simulink model "torqueWalkingR2012b"  (Simulink 8.0)
settings: Solver=FixedStepDiscrete  StartTime=0.0  StopTime=Config.t_end  FixedStep=Config.t_step  RelTol=1e-3
InitFcn:
  | cd(fileparts(which(bdroot)));
  | initTorqueWalking;
StopFcn:
  | disp_early_termination
undefined symbols (not defined in the file or in its folder): biasVectorConstraint_feet, Config, ConstraintMatrix_feet, DiscIntNeverNeededParam, Gains, ROBOT_DOF, Sat
libraries: WBToolboxLibrary x114, simulink x2
(part 1 of 4)
settings Model: Creator=gnava  LastModifiedBy=mcharbonneau
settings DataIOCC: LimitDataPoints=off  SaveFormat=StructureWithTime
settings OptimizationCC: ExpressionDepthLimit=128
settings DebuggingCC: UnderspecifiedInitializationDetection=Simplified  MergeDetectMultiDrivingBlocksExec=error  SolverPrmCheckMsg=none  InheritedTsInSrcMsg=none  UnconnectedLineMsg=none  FrameProcessingCompatibilityMsg=error  StateNameClashWarn=none  SFUnexpectedBacktrackingDiag=error  SFNoUnconditionalDefaultTransitionDiag=error
settings HardwareCC: ProdBitPerPointer=64  ProdLargestAtomicFloat=Float  ProdIntDivRoundTo=Zero  ProdEndianess=LittleEndian  ProdHWDeviceType=Specified
settings ModelReferenceCC: PropagateSignalLabelsOutOfModel=on
settings CodeAppCC: CustomSymbolStrType=$N$R$M_T
settings GRTTargetCC: CodeReplacementLibrary=C99 (ISO)  GeneratePreprocessorConditionals=Use local settings

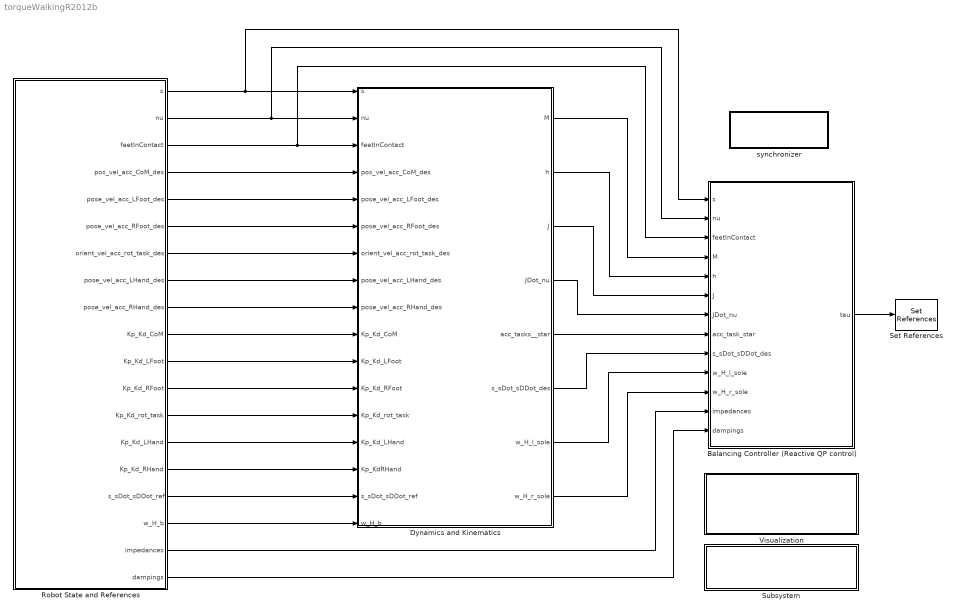
== system torqueWalkingR2012b ==
  Balancing Controller (Reactive QP control) : Subsystem
  Dynamics and Kinematics : Subsystem
  Robot State and References : Subsystem
  Set References : WBToolboxLibrary/wholeBodyActuators/Set References  controlType=Torque  fullOrSubControl=Full  controlledJoints=''  robotName=WBT_robotName  localName=WBT_modelName  wbiFile=WBT_wbiFilename  wbiList=WBT_wbiList
  Subsystem : Subsystem
      mask Display: disp('DATA FOR LEARNOPTIM_WBC')
  Visualization : Subsystem
      mask Display: disp('VISUALIZE AND DUMP DATA \n EARLY TERMINATION')
  synchronizer : Subsystem
      mask Display: disp('SYNCHRONIZER')
  wires:
  Robot State and References/2(nu) -> Dynamics and Kinematics/2(nu), Balancing Controller (Reactive QP control)/2(nu)
  Robot State and References/3(feetInContact) -> Dynamics and Kinematics/3(feetInContact), Balancing Controller (Reactive QP control)/3(feetInContact)
  Robot State and References/4(pos_vel_acc_CoM_des) -> Dynamics and Kinematics/4(pos_vel_acc_CoM_des)
  Robot State and References/5(pose_vel_acc_LFoot_des) -> Dynamics and Kinematics/5(pose_vel_acc_LFoot_des)
  Robot State and References/6(pose_vel_acc_RFoot_des) -> Dynamics and Kinematics/6(pose_vel_acc_RFoot_des)
  Robot State and References/11(Kp_Kd_LFoot) -> Dynamics and Kinematics/11(Kp_Kd_LFoot)
  Robot State and References/12(Kp_Kd_RFoot) -> Dynamics and Kinematics/12(Kp_Kd_RFoot)
  Robot State and References/13(Kp_Kd_rot_task) -> Dynamics and Kinematics/13(Kp_Kd_rot_task)
  Robot State and References/16(s_sDot_sDDot_ref) -> Dynamics and Kinematics/16(s_sDot_sDDot_ref)
  Robot State and References/17(w_H_b) -> Dynamics and Kinematics/17(w_H_b)
  Dynamics and Kinematics/4(JDot_nu) -> Balancing Controller (Reactive QP control)/7(JDot_nu)
  Robot State and References/1(s) -> Dynamics and Kinematics/1(s), Balancing Controller (Reactive QP control)/1(s)
  Dynamics and Kinematics/1(M) -> Balancing Controller (Reactive QP control)/4(M)
  Dynamics and Kinematics/2(h) -> Balancing Controller (Reactive QP control)/5(h)
  Dynamics and Kinematics/3(J) -> Balancing Controller (Reactive QP control)/6(J)
  Balancing Controller (Reactive QP control)/1(tau) -> Set References/1
  Dynamics and Kinematics/5(acc_tasks__star) -> Balancing Controller (Reactive QP control)/8(acc_task_star)
  Dynamics and Kinematics/6(s_sDot_sDDot_des) -> Balancing Controller (Reactive QP control)/9(s_sDot_sDDot_des)
  Dynamics and Kinematics/7(w_H_l_sole) -> Balancing Controller (Reactive QP control)/10(w_H_l_sole)
  Dynamics and Kinematics/8(w_H_r_sole) -> Balancing Controller (Reactive QP control)/11(w_H_r_sole)
  Robot State and References/18(impedances) -> Balancing Controller (Reactive QP control)/12(impedances)
  Robot State and References/19(dampings) -> Balancing Controller (Reactive QP control)/13(dampings)
  Robot State and References/15(Kp_Kd_RHand) -> Dynamics and Kinematics/15(Kp_KdRHand)
  Robot State and References/14(Kp_Kd_LHand) -> Dynamics and Kinematics/14(Kp_Kd_LHand)
  Robot State and References/8(pose_vel_acc_LHand_des) -> Dynamics and Kinematics/8(pose_vel_acc_LHand_des)
  Robot State and References/7(orient_vel_acc_rot_task_des) -> Dynamics and Kinematics/7(orient_vel_acc_rot_task_des)
  Robot State and References/9(pose_vel_acc_RHand_des) -> Dynamics and Kinematics/9(pose_vel_acc_RHand_des)
  Robot State and References/10(Kp_Kd_CoM) -> Dynamics and Kinematics/10(Kp_Kd_CoM)

== system torqueWalkingR2012b/Balancing Controller (Reactive QP control) ==
  s : Inport
  nu : Inport  Port=2
  feetInContact : Inport  Port=3
  M : Inport  Port=4
  h : Inport  Port=5
  J : Inport  Port=6
  JDot_nu : Inport  Port=7
  acc_task_star : Inport  Port=8
  s_sDot_sDDot_des : Inport  Port=9
  w_H_l_sole : Inport  Port=10
  w_H_r_sole : Inport  Port=11
  impedances : Inport  Port=12
  dampings : Inport  Port=13
  "   " : Constant  Value=ConstraintMatrix_feet
  "      " : Constant  Value=biasVectorConstraint_feet
  "             " : Selector  InputPortWidth=ROBOT_DOF+6  IndexOptions=Index vector (dialog)  Indices=[7:ROBOT_DOF+6]  OutputSizes=1
  Balancing Controller Function : MATLAB Function  TreatAsAtomicUnit=on
      settings: PermitHierarchicalResolution=ParametersOnly
  Compute joint torques (motor reflected inertia) : Subsystem
  Get Estimate : WBToolboxLibrary/wholeBodyStates/Get Estimate  estimateType=Joints Torque  robotName=WBT_robotName  localName=WBT_modelName  wbiFile=WBT_wbiFilename  wbiList=WBT_wbiList
  QPSolver (Reactive QP control) : Subsystem
  Saturation : Saturate  UpperLimit=Sat.tau_max  LowerLimit=-Sat.tau_max
  "holder " : WBToolboxLibrary/Utilities/holder 
  tau : Outport
  tag scope: exitFlagQP=global, f_LFoot=global, f_RFoot=global, tau=global, tau_des=global
  wires:
  QPSolver (Reactive QP control)/1(tau) -> Compute joint torques (motor reflected inertia)/1(invGamma*tau_motors)
  "holder "/1 -> QPSolver (Reactive QP control)/1(tau_0)
  Balancing Controller Function/3(ConstraintMatrix_equality) -> QPSolver (Reactive QP control)/5(ConstraintMatrix_equality)
  Balancing Controller Function/6(biasVectorConstraint_inequality) -> QPSolver (Reactive QP control)/8(biasVectorConstraint_inequality)
  Balancing Controller Function/2(gradient) -> QPSolver (Reactive QP control)/4(gradient)
  Balancing Controller Function/4(biasVectorConstraint_equality) -> QPSolver (Reactive QP control)/6(biasVectorConstraint_equality)
  Balancing Controller Function/5(ConstraintMatrix_inequality) -> QPSolver (Reactive QP control)/7(ConstraintMatrix_inequality)
  w_H_r_sole/1 -> Balancing Controller Function/15(w_H_r_sole)
  w_H_l_sole/1 -> Balancing Controller Function/14(w_H_l_sole)
  "      "/1 -> Balancing Controller Function/13(biasVectorConstraint_feet)
  "   "/1 -> Balancing Controller Function/12(ConstraintsMatrix_feet)
  s_sDot_sDDot_des/1 -> Balancing Controller Function/9(s_sDot_sDDot_des)
  nu/1 -> "             "/1
  s/1 -> Balancing Controller Function/7(s)
  dampings/1 -> Balancing Controller Function/6(dampings)
  impedances/1 -> Balancing Controller Function/5(impedances)
  h/1 -> Balancing Controller Function/3(h)
  M/1 -> Balancing Controller Function/2(M)
  Get Estimate/1 -> [tau], "holder "/1
  "             "/1 -> Balancing Controller Function/8(sDot)
  Saturation/1 -> tau/1, [tau_des]
  Balancing Controller Function/1(Hessian) -> QPSolver (Reactive QP control)/3(Hessian)
  feetInContact/1 -> QPSolver (Reactive QP control)/2(feetInContact), Balancing Controller Function/1(feetInContact)
  QPSolver (Reactive QP control)/2(f_LFoot) -> [f_LFoot]
  QPSolver (Reactive QP control)/3(f_RFoot) -> [f_RFoot]
  QPSolver (Reactive QP control)/4(exitFlagQP) -> [exitFlagQP]
  Compute joint torques (motor reflected inertia)/1(tau_joints) -> Saturation/1
  acc_task_star/1 -> Balancing Controller Function/10(acc_task_star)
  J/1 -> Balancing Controller Function/4(J)
  JDot_nu/1 -> Balancing Controller Function/11(JDot_nu)

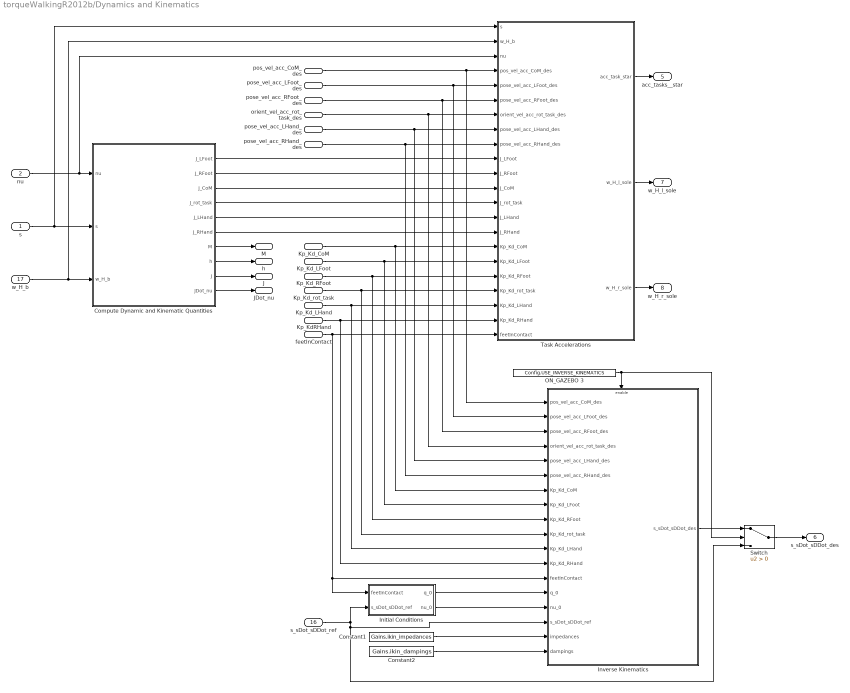
== system torqueWalkingR2012b/Dynamics and Kinematics ==
  s : Inport
  nu : Inport  Port=2
  feetInContact : Inport  Port=3
  pos_vel_acc_CoM_des : Inport  Port=4
  pose_vel_acc_LFoot_des : Inport  Port=5
  pose_vel_acc_RFoot_des : Inport  Port=6
  orient_vel_acc_rot_task_des : Inport  Port=7
  pose_vel_acc_LHand_des : Inport  Port=8
  pose_vel_acc_RHand_des : Inport  Port=9
  Kp_Kd_CoM : Inport  Port=10
  Kp_Kd_LFoot : Inport  Port=11
  Kp_Kd_RFoot : Inport  Port=12
  Kp_Kd_rot_task : Inport  Port=13
  Kp_Kd_LHand : Inport  Port=14
  Kp_KdRHand : Inport  Port=15
  s_sDot_sDDot_ref : Inport  Port=16
  w_H_b : Inport  Port=17
  Compute Dynamic and Kinematic Quantities : Subsystem
  Constant1 : Constant  Value=Gains.ikin_impedances
  Constant2 : Constant  Value=Gains.ikin_dampings
  Initial Conditions : Subsystem
  Inverse Kinematics : Subsystem
  ON_GAZEBO 3 : Constant  Value=Config.USE_INVERSE_KINEMATICS
  Switch : Switch  Criteria=u2 > Threshold
  Task Accelerations : Subsystem
  M : Outport
  h : Outport  Port=2
  J : Outport  Port=3
  JDot_nu : Outport  Port=4
  acc_tasks__star : Outport  Port=5
  s_sDot_sDDot_des : Outport  Port=6
  w_H_l_sole : Outport  Port=7
  w_H_r_sole : Outport  Port=8
  wires:
  pos_vel_acc_CoM_des/1 -> Inverse Kinematics/1(pos_vel_acc_CoM_des), Task Accelerations/4(pos_vel_acc_CoM_des)
  pose_vel_acc_LFoot_des/1 -> Inverse Kinematics/2(pose_vel_acc_LFoot_des), Task Accelerations/5(pose_vel_acc_LFoot_des)
  pose_vel_acc_RFoot_des/1 -> Inverse Kinematics/3(pose_vel_acc_RFoot_des), Task Accelerations/6(pose_vel_acc_RFoot_des)
  orient_vel_acc_rot_task_des/1 -> Inverse Kinematics/4(orient_vel_acc_rot_task_des), Task Accelerations/7(orient_vel_acc_rot_task_des)
  Kp_Kd_CoM/1 -> Inverse Kinematics/7(Kp_Kd_CoM), Task Accelerations/16(Kp_Kd_CoM)
  Kp_Kd_LFoot/1 -> Inverse Kinematics/8(Kp_Kd_LFoot), Task Accelerations/17(Kp_Kd_LFoot)
  Kp_Kd_RFoot/1 -> Inverse Kinematics/9(Kp_Kd_RFoot), Task Accelerations/18(Kp_Kd_RFoot)
  Kp_Kd_rot_task/1 -> Inverse Kinematics/10(Kp_Kd_rot_task), Task Accelerations/19(Kp_Kd_rot_task)
  Task Accelerations/1(acc_task_star) -> acc_tasks__star/1
  ON_GAZEBO 3/1 -> Switch/2, Inverse Kinematics/Enable
  Inverse Kinematics/1(s_sDot_sDDot_des) -> Switch/1
  nu/1 -> Task Accelerations/3(nu), Compute Dynamic and Kinematic Quantities/1(nu)
  s/1 -> Task Accelerations/1(s), Compute Dynamic and Kinematic Quantities/2(s)
  w_H_b/1 -> Task Accelerations/2(w_H_b), Compute Dynamic and Kinematic Quantities/3(w_H_b)
  Compute Dynamic and Kinematic Quantities/8(h) -> h/1
  Compute Dynamic and Kinematic Quantities/1(J_LFoot) -> Task Accelerations/10(J_LFoot)
  Compute Dynamic and Kinematic Quantities/2(J_RFoot) -> Task Accelerations/11(J_RFoot)
  Compute Dynamic and Kinematic Quantities/3(J_CoM) -> Task Accelerations/12(J_CoM)
  Compute Dynamic and Kinematic Quantities/7(M) -> M/1
  Compute Dynamic and Kinematic Quantities/4(J_rot_task) -> Task Accelerations/13(J_rot_task)
  Compute Dynamic and Kinematic Quantities/9(J) -> J/1
  Compute Dynamic and Kinematic Quantities/10(JDot_nu) -> JDot_nu/1
  s_sDot_sDDot_ref/1 -> Inverse Kinematics/16(s_sDot_sDDot_ref), Switch/3, Initial Conditions/2(s_sDot_sDDot_ref)
  Initial Conditions/1(q_0) -> Inverse Kinematics/14(q_0)
  Initial Conditions/2(nu_0) -> Inverse Kinematics/15(nu_0)
  Constant1/1 -> Inverse Kinematics/17(impedances)
  Constant2/1 -> Inverse Kinematics/18(dampings)
  Switch/1 -> s_sDot_sDDot_des/1
  feetInContact/1 -> Task Accelerations/22(feetInContact), Inverse Kinematics/13(feetInContact), Initial Conditions/1(feetInContact)
  Task Accelerations/2(w_H_l_sole) -> w_H_l_sole/1
  Task Accelerations/3(w_H_r_sole) -> w_H_r_sole/1
  Compute Dynamic and Kinematic Quantities/5(J_LHand) -> Task Accelerations/14(J_LHand)
  Compute Dynamic and Kinematic Quantities/6(J_RHand) -> Task Accelerations/15(J_RHand)
  pose_vel_acc_RHand_des/1 -> Inverse Kinematics/6(pose_vel_acc_RHand_des), Task Accelerations/9(pose_vel_acc_RHand_des)
  pose_vel_acc_LHand_des/1 -> Inverse Kinematics/5(pose_vel_acc_LHand_des), Task Accelerations/8(pose_vel_acc_LHand_des)
  Kp_Kd_LHand/1 -> Inverse Kinematics/11(Kp_Kd_LHand), Task Accelerations/20(Kp_Kd_LHand)
  Kp_KdRHand/1 -> Inverse Kinematics/12(Kp_Kd_RHand), Task Accelerations/21(Kp_Kd_RHand)

== system torqueWalkingR2012b/Robot State and References ==
  Gain Scheduling : Subsystem
  "Smooth References " : Subsystem
  State Machines : Subsystem
  s : Outport
  nu : Outport  Port=2
  feetInContact : Outport  Port=3
  pos_vel_acc_CoM_des : Outport  Port=4
  pose_vel_acc_LFoot_des : Outport  Port=5
  pose_vel_acc_RFoot_des : Outport  Port=6
  orient_vel_acc_rot_task_des : Outport  Port=7
  pose_vel_acc_LHand_des : Outport  Port=8
  pose_vel_acc_RHand_des : Outport  Port=9
  Kp_Kd_CoM : Outport  Port=10
  Kp_Kd_LFoot : Outport  Port=11
  Kp_Kd_RFoot : Outport  Port=12
  Kp_Kd_rot_task : Outport  Port=13
  Kp_Kd_LHand : Outport  Port=14
  Kp_Kd_RHand : Outport  Port=15
  s_sDot_sDDot_ref : Outport  Port=16
  w_H_b : Outport  Port=17
  impedances : Outport  Port=18
  dampings : Outport  Port=19
  wires:
  Gain Scheduling/1(Kp_Kd_CoM) -> Kp_Kd_CoM/1
  Gain Scheduling/2(Kp_Kd_LFoot) -> Kp_Kd_LFoot/1
  Gain Scheduling/3(Kp_Kd_RFoot) -> Kp_Kd_RFoot/1
  Gain Scheduling/4(Kp_Kd_rot_task) -> Kp_Kd_rot_task/1
  Gain Scheduling/7(impedances) -> impedances/1
  Gain Scheduling/8(dampings) -> dampings/1
  State Machines/5(state) -> Gain Scheduling/1(state), "Smooth References "/1(state)
  State Machines/4(feetInContact) -> feetInContact/1
  State Machines/3(nu) -> nu/1
  State Machines/2(w_H_b) -> w_H_b/1
  State Machines/8(references_CoM) -> "Smooth References "/4(references_CoM)
  State Machines/6(references_LFoot) -> "Smooth References "/2(references_LFoot)
  State Machines/7(references_RFoot) -> "Smooth References "/3(references_RFoot)
  State Machines/9(references_rot_task) -> "Smooth References "/5(references_rot_task)
  State Machines/12(references_s) -> "Smooth References "/8(references_s)
  "Smooth References "/1(pos_vel_acc_CoM_des) -> pos_vel_acc_CoM_des/1
  "Smooth References "/2(pose_vel_acc_LFoot_des) -> pose_vel_acc_LFoot_des/1
  "Smooth References "/3(pose_vel_acc_RFoot_des) -> pose_vel_acc_RFoot_des/1
  "Smooth References "/4(orient_vel_acc_rot_task_des) -> orient_vel_acc_rot_task_des/1
  "Smooth References "/7(s_sDot_sDDot_ref) -> s_sDot_sDDot_ref/1
  State Machines/1(s) -> s/1
  State Machines/10(references_LHand) -> "Smooth References "/6(references_LHand)
  State Machines/11(references_RHand) -> "Smooth References "/7(references_RHand)
  "Smooth References "/5(pose_vel_acc_LHand_des) -> pose_vel_acc_LHand_des/1
  "Smooth References "/6(pose_vel_acc_RHand_des) -> pose_vel_acc_RHand_des/1
  Gain Scheduling/5(Kp_Kd_LHand) -> Kp_Kd_LHand/1
  Gain Scheduling/6(Kp_Kd_RHand) -> Kp_Kd_RHand/1

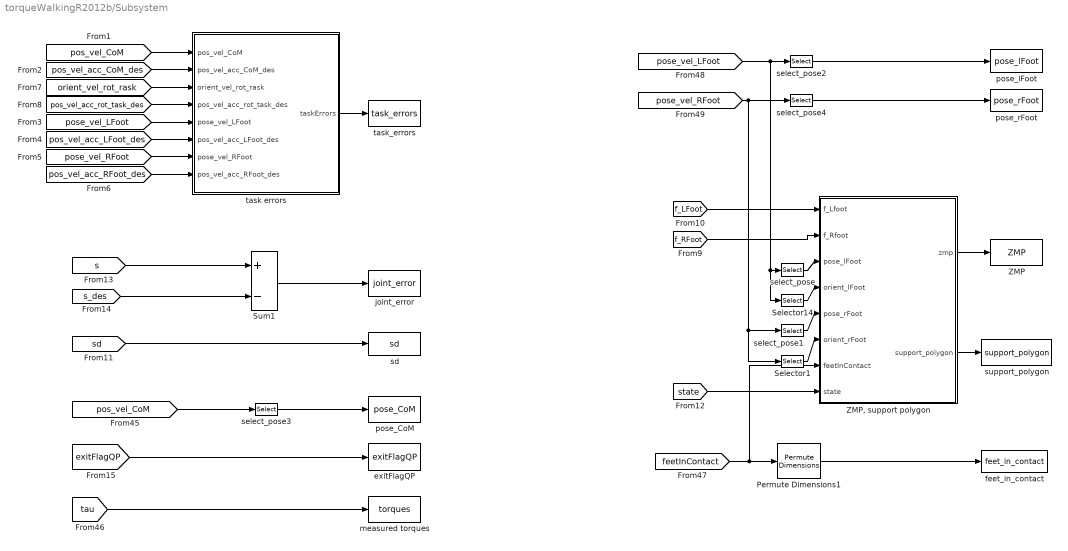
== system torqueWalkingR2012b/Subsystem ==
  Permute Dimensions1 : PermuteDimensions
  Selector1 : Selector  NumberOfDimensions=2  InputPortWidth=3  IndexOptions=Index vector (dialog),Index vector (dialog)  Indices=[4:6],[1:3]  OutputSizes=1,1
  Selector14 : Selector  NumberOfDimensions=2  InputPortWidth=3  IndexOptions=Index vector (dialog),Index vector (dialog)  Indices=[4:6],[1:3]  OutputSizes=1,1
  Sum1 : Sum  Inputs=+-
  ZMP : ToWorkspace  VariableName=ZMP  SaveFormat=Timeseries  SampleTime=-1
  "ZMP, support polygon" : Subsystem
  exitFlagQP : ToWorkspace  VariableName=exitFlagQP  SaveFormat=Timeseries  SampleTime=-1
  feet_in_contact : ToWorkspace  VariableName=feet_in_contact  SaveFormat=Timeseries  SampleTime=-1
  joint_error : ToWorkspace  VariableName=joint_error  SaveFormat=Timeseries  SampleTime=-1
  measured torques : ToWorkspace  VariableName=torques  SaveFormat=Timeseries  SampleTime=-1
  pose_CoM : ToWorkspace  VariableName=pose_CoM  SaveFormat=Timeseries  SampleTime=-1
  pose_lFoot : ToWorkspace  VariableName=pose_lFoot  SaveFormat=Timeseries  SampleTime=-1
  pose_rFoot : ToWorkspace  VariableName=pose_rFoot  SaveFormat=Timeseries  SampleTime=-1
  sd : ToWorkspace  VariableName=sd  SaveFormat=Timeseries  SampleTime=-1
  select_pose{,1..4} (5 alike) : Selector  NumberOfDimensions=2  InputPortWidth=3  IndexOptions=Index vector (dialog),Index vector (dialog)  Indices=[1:3],1  OutputSizes=1,1
  support_polygon : ToWorkspace  VariableName=support_polygon  SaveFormat=Timeseries  SampleTime=-1
  task errors : Subsystem
  task_errors : ToWorkspace  VariableName=task_errors  SaveFormat=Timeseries  SampleTime=-1
  wires:
  select_pose4/1 -> pose_rFoot/1
  [s_des] -> Sum1/2
  select_pose2/1 -> pose_lFoot/1
  select_pose3/1 -> pose_CoM/1
  [pos_vel_CoM] -> select_pose3/1
  [s] -> Sum1/1
  [exitFlagQP] -> exitFlagQP/1
  [sd] -> sd/1
  Sum1/1 -> joint_error/1
  [pose_vel_LFoot] -> Selector14/1, select_pose/1, select_pose2/1
  [feetInContact] -> Permute Dimensions1/1, "ZMP, support polygon"/7(feetInContact)
  [tau] -> measured torques/1
  Permute Dimensions1/1 -> feet_in_contact/1
  [pos_vel_CoM] -> task errors/1(pos_vel_CoM)
  [pos_vel_acc_CoM_des] -> task errors/2(pos_vel_acc_CoM_des)
  [orient_vel_rot_rask] -> task errors/3(orient_vel_rot_rask)
  [pos_vel_acc_rot_task_des] -> task errors/4(pos_vel_acc_rot_task_des)
  [pose_vel_LFoot] -> task errors/5(pose_vel_LFoot)
  [pos_vel_acc_LFoot_des] -> task errors/6(pos_vel_acc_LFoot_des)
  [pose_vel_RFoot] -> task errors/7(pose_vel_RFoot)
  [pos_vel_acc_RFoot_des] -> task errors/8(pos_vel_acc_RFoot_des)
  Selector14/1 -> "ZMP, support polygon"/4(orient_lFoot)
  select_pose1/1 -> "ZMP, support polygon"/5(pose_rFoot)
  select_pose/1 -> "ZMP, support polygon"/3(pose_lFoot)
  "ZMP, support polygon"/1(zmp) -> ZMP/1
  Selector1/1 -> "ZMP, support polygon"/6(orient_rFoot)
  [pose_vel_RFoot] -> Selector1/1, select_pose1/1, select_pose4/1
  [f_LFoot] -> "ZMP, support polygon"/1(f_Lfoot)
  [f_RFoot] -> "ZMP, support polygon"/2(f_Rfoot)
  "ZMP, support polygon"/2(support_polygon) -> support_polygon/1
  task errors/1(taskErrors) -> task_errors/1
  [state] -> "ZMP, support polygon"/8(state)

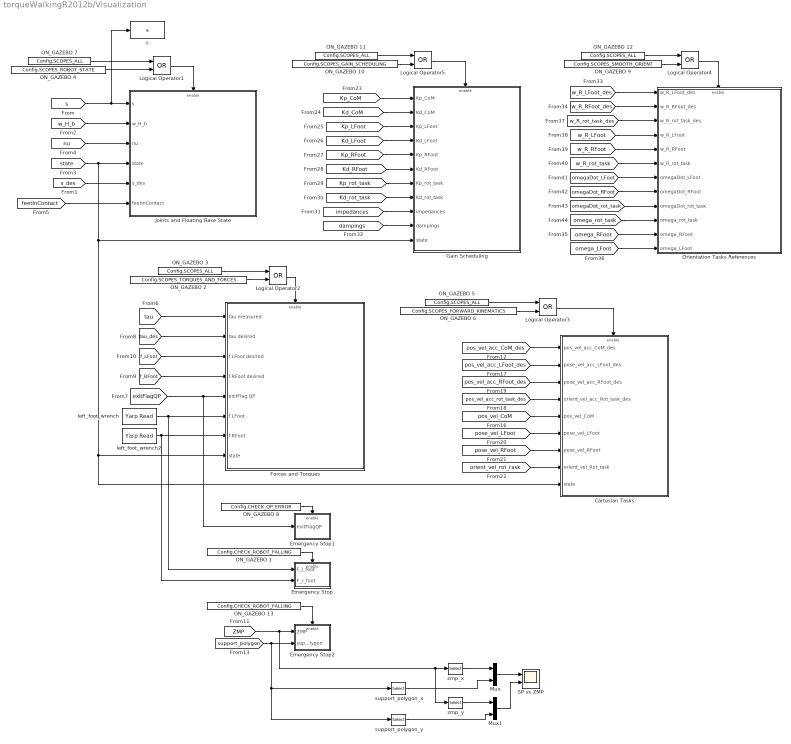
== system torqueWalkingR2012b/Visualization ==
  Cartesian Tasks : Subsystem
  Emergency Stop : Subsystem
  Emergency Stop1 : Subsystem
  Emergency Stop2 : Subsystem
  Forces and Torques : Subsystem
  Gain Scheduling : Subsystem
  Joints and Floating Base State : Subsystem
  Logical Operator{1..5} (5 alike) : Logic  Operator=OR  AllPortsSameDT=off  OutDataTypeStr=boolean
  Mux : Mux  Inputs=2
  Mux1 : Mux  Inputs=2
  ON_GAZEBO 1 : Constant  Value=Config.CHECK_ROBOT_FALLING
  ON_GAZEBO 10 : Constant  Value=Config.SCOPES_GAIN_SCHEDULING
  ON_GAZEBO {3,5,7,11..12} (5 alike) : Constant  Value=Config.SCOPES_ALL
  ON_GAZEBO 13 : Constant  Value=Config.CHECK_ROBOT_FALLING
  ON_GAZEBO 2 : Constant  Value=Config.SCOPES_TORQUES_AND_FORCES
  ON_GAZEBO 4 : Constant  Value=Config.SCOPES_ROBOT_STATE
  ON_GAZEBO 6 : Constant  Value=Config.SCOPES_FORWARD_KINEMATICS
  ON_GAZEBO 8 : Constant  Value=Config.CHECK_QP_ERROR
  ON_GAZEBO 9 : Constant  Value=Config.SCOPES_SMOOTH_ORIENT
  Orientation Tasks References : Subsystem
  SP vs ZMP : Scope  NumInputPorts=2
      settings: TimeRange=auto  MaxDataPoints=5000  SaveToWorkspace=off  YMin=-0.07444~-0.1845  YMax=0.11943~0.04889  SampleTime=-1
  left_foot_wrench : WBToolboxLibrary/Utilities/Yarp Read  portName=Ports.LEFT_FOOT_EXT_WRENCH  signalSize=6  blocking=off  timestamp=off  autoconnect=on  errorOnConnection=on
  left_foot_wrench2 : WBToolboxLibrary/Utilities/Yarp Read  portName=Ports.RIGHT_FOOT_EXT_WRENCH  signalSize=6  blocking=off  timestamp=off  autoconnect=on  errorOnConnection=on
  s : ToWorkspace  VariableName=s  SaveFormat=Timeseries  SampleTime=-1
  support_polygon_x : Selector  NumberOfDimensions=2  InputPortWidth=6  IndexOptions=Index vector (dialog),Index vector (dialog)  Indices=1,[1 2]  OutputSizes=1,1
  support_polygon_y : Selector  NumberOfDimensions=2  InputPortWidth=6  IndexOptions=Index vector (dialog),Index vector (dialog)  Indices=2,[1 2]  OutputSizes=1,1
  zmp_x : Selector  NumberOfDimensions=2  InputPortWidth=6  IndexOptions=Index vector (dialog),Index vector (dialog)  Indices=1,1  OutputSizes=1,1
  zmp_y : Selector  NumberOfDimensions=2  InputPortWidth=6  IndexOptions=Index vector (dialog),Index vector (dialog)  Indices=1,2  OutputSizes=1,1
  wires:
  [s] -> s/1, Joints and Floating Base State/1(s)
  [w_H_b] -> Joints and Floating Base State/2(w_H_b)
  [s_des] -> Joints and Floating Base State/5(s_des)
  [nu] -> Joints and Floating Base State/3(nu)
  [state] -> Cartesian Tasks/9(state), Forces and Torques/8(state), Gain Scheduling/11(state), Joints and Floating Base State/4(state)
  [tau] -> Forces and Torques/1(tau measured)
  [tau_des] -> Forces and Torques/2(tau desired)
  [f_LFoot] -> Forces and Torques/3(f LFoot desired)
  [f_RFoot] -> Forces and Torques/4(f RFoot desired)
  ON_GAZEBO 4/1 -> Logical Operator1/2
  ON_GAZEBO 7/1 -> Logical Operator1/1
  Logical Operator1/1 -> Joints and Floating Base State/Enable
  [feetInContact] -> Joints and Floating Base State/6(feetInContact)
  Logical Operator2/1 -> Forces and Torques/Enable
  ON_GAZEBO 3/1 -> Logical Operator2/1
  ON_GAZEBO 2/1 -> Logical Operator2/2
  ON_GAZEBO 6/1 -> Logical Operator3/2
  Logical Operator3/1 -> Cartesian Tasks/Enable
  ON_GAZEBO 5/1 -> Logical Operator3/1
  [pos_vel_acc_CoM_des] -> Cartesian Tasks/1(pos_vel_acc_CoM_des)
  [pos_vel_acc_LFoot_des] -> Cartesian Tasks/2(pose_vel_acc_LFoot_des)
  [pos_vel_acc_RFoot_des] -> Cartesian Tasks/3(pose_vel_acc_RFoot_des)
  [pos_vel_acc_rot_task_des] -> Cartesian Tasks/4(orient_vel_acc_Rot_task_des)
  [pos_vel_CoM] -> Cartesian Tasks/5(pos_vel_CoM)
  [pose_vel_LFoot] -> Cartesian Tasks/6(pose_vel_LFoot)
  [pose_vel_RFoot] -> Cartesian Tasks/7(pose_vel_RFoot)
  [orient_vel_rot_rask] -> Cartesian Tasks/8(orient_vel_Rot_task)
  ON_GAZEBO 10/1 -> Logical Operator5/2
  ON_GAZEBO 11/1 -> Logical Operator5/1
  Logical Operator5/1 -> Gain Scheduling/Enable
  [Kp_CoM] -> Gain Scheduling/1(Kp_CoM)
  [Kd_CoM] -> Gain Scheduling/2(Kd_CoM)
  [Kp_LFoot] -> Gain Scheduling/3(Kp_LFoot)
  [Kd_LFoot] -> Gain Scheduling/4(Kd_LFoot)
  [Kp_RFoot] -> Gain Scheduling/5(Kp_RFoot)
  [Kd_RFoot] -> Gain Scheduling/6(Kd_RFoot)
  [Kp_rot_task] -> Gain Scheduling/7(Kp_rot_task)
  [Kd_rot_task] -> Gain Scheduling/8(Kd_rot_task)
  [impedances] -> Gain Scheduling/9(impedances)
  [dampings] -> Gain Scheduling/10(dampings)
  ON_GAZEBO 9/1 -> Logical Operator4/2
  ON_GAZEBO 12/1 -> Logical Operator4/1
  Logical Operator4/1 -> Orientation Tasks References/Enable
  [omega_LFoot] -> Orientation Tasks References/12(omega_LFoot)
  [omega_RFoot] -> Orientation Tasks References/11(omega_RFoot)
  [omega_rot_task] -> Orientation Tasks References/10(omega_rot_task)
  [omegaDot_RFoot] -> Orientation Tasks References/8(omegaDot_RFoot)
  [omegaDot_rot_task] -> Orientation Tasks References/9(omegaDot_rot_task)
  [omegaDot_LFoot] -> Orientation Tasks References/7(omegaDot_LFoot)
  [w_R_LFoot_des] -> Orientation Tasks References/1(w_R_LFoot_des)
  [w_R_RFoot_des] -> Orientation Tasks References/2(w_R_RFoot_des)
  [w_R_rot_task_des] -> Orientation Tasks References/3(w_R_rot_task_des)
  [w_R_LFoot] -> Orientation Tasks References/4(w_R_LFoot)
  [w_R_RFoot] -> Orientation Tasks References/5(w_R_RFoot)
  [w_R_rot_task] -> Orientation Tasks References/6(w_R_rot_task)
  ON_GAZEBO 1/1 -> Emergency Stop/Enable
  [exitFlagQP] -> Emergency Stop1/1(exitFlagQP), Forces and Torques/5(exitFlag QP)
  ON_GAZEBO 8/1 -> Emergency Stop1/Enable
  left_foot_wrench/1 -> Emergency Stop/1(F_l_foot), Forces and Torques/6(f LFoot)
  left_foot_wrench2/1 -> Forces and Torques/7(f RFoot), Emergency Stop/2(F_r_foot)
  ON_GAZEBO 13/1 -> Emergency Stop2/Enable
  [ZMP] -> zmp_y/1, zmp_x/1, Emergency Stop2/1(ZMP)
  zmp_y/1 -> Mux1/1
  [support_polygon] -> support_polygon_y/1, support_polygon_x/1, Emergency Stop2/2(support_polygon)
  support_polygon_x/1 -> Mux/2
  Mux1/1 -> SP vs ZMP/2
  Mux/1 -> SP vs ZMP/1
  zmp_x/1 -> Mux/1
  support_polygon_y/1 -> Mux1/2

== system torqueWalkingR2012b/synchronizer ==
  GAZEBO_SYNCHRONIZER : Subsystem
  Logical Operator : Logic  Operator=NOT  AllPortsSameDT=off  OutDataTypeStr=boolean
  "ON_GAZEBO " : Constant  Value=Config.ON_GAZEBO
  REAL_TIME_SYNC : Subsystem
  wires:
  Logical Operator/1 -> REAL_TIME_SYNC/Enable
  "ON_GAZEBO "/1 -> Logical Operator/1, GAZEBO_SYNCHRONIZER/Enable

== system torqueWalkingR2012b/Balancing Controller (Reactive QP control)/Compute joint torques (motor reflected inertia) ==
  invGamma*tau_motors : Inport
  " " : Constant  Value=Config.USE_MOTOR_REFLECTED_INERTIA
  Add : Sum  Inputs=-+
  Gain : Gain  Gain=Config.K_ff
  Get Estimate : WBToolboxLibrary/wholeBodyStates/Get Estimate  estimateType=Joints Acceleration  robotName=WBT_robotName  localName=WBT_modelName  wbiFile=WBT_wbiFilename  wbiList=WBT_wbiList
  Motors Inertia : Constant  Value=Config.I_m
  Product : Product  Multiplication=Matrix(*)
  Product1 : Product  Multiplication=Matrix(*)
  Switch : Switch  Criteria=u2 > Threshold
  Transmission ratio : Constant  Value=Config.invGamma
  tau_joints : Outport
  wires:
  Product1/1 -> Product/1
  Get Estimate/1 -> Product/2
  Product/1 -> Gain/1
  Transmission ratio/1 -> Product1/1
  Motors Inertia/1 -> Product1/2
  Gain/1 -> Add/1
  Add/1 -> Switch/1
  " "/1 -> Switch/2
  Switch/1 -> tau_joints/1
  invGamma*tau_motors/1 -> Switch/3, Add/2

== system torqueWalkingR2012b/Balancing Controller (Reactive QP control)/QPSolver (Reactive QP control) ==
  tau_0 : Inport
  feetInContact : Inport  Port=2
  Hessian : Inport  Port=3
  gradient : Inport  Port=4
  ConstraintMatrix_equality : Inport  Port=5
  biasVectorConstraint_equality : Inport  Port=6
  ConstraintMatrix_inequality : Inport  Port=7
  biasVectorConstraint_inequality : Inport  Port=8
  QPSolver : M-S-Function  FunctionName=QPBalancing  Parameters=ROBOT_DOF, Sat, Config
  tau : Outport
  f_LFoot : Outport  Port=2
  f_RFoot : Outport  Port=3
  exitFlagQP : Outport  Port=4
  wires:
  gradient/1 -> QPSolver/4
  Hessian/1 -> QPSolver/3
  biasVectorConstraint_inequality/1 -> QPSolver/8
  feetInContact/1 -> QPSolver/2
  QPSolver/2 -> f_LFoot/1
  ConstraintMatrix_inequality/1 -> QPSolver/7
  biasVectorConstraint_equality/1 -> QPSolver/6
  ConstraintMatrix_equality/1 -> QPSolver/5
  tau_0/1 -> QPSolver/1
  QPSolver/1 -> tau/1
  QPSolver/3 -> f_RFoot/1
  QPSolver/4 -> exitFlagQP/1

== system torqueWalkingR2012b/Dynamics and Kinematics/Compute Dynamic and Kinematic Quantities ==
  nu : Inport
  s : Inport  Port=2
  w_H_b : Inport  Port=3
  "  " : Selector  NumberOfDimensions=2  InputPortWidth=ROBOT_DOF+16  IndexOptions=Index vector (dialog),Index vector (dialog)  Indices=[1:3],[1:ROBOT_DOF+6]  OutputSizes=1,1
  "   " : Selector  InputPortWidth=6  IndexOptions=Index vector (dialog)  Indices=[1:3]  OutputSizes=1
  "     " : Selector  NumberOfDimensions=2  InputPortWidth=ROBOT_DOF+16  IndexOptions=Index vector (dialog),Index vector (dialog)  Indices=[4:6],[1:ROBOT_DOF+6]  OutputSizes=1,1
  "               " : Selector  InputPortWidth=6  IndexOptions=Index vector (dialog)  Indices=[4:6]  OutputSizes=1
  Jacobians and JDot_nu : Subsystem
  Mass Matrix and Bias Forces : Subsystem
  Matrix Concatenate : Concatenate  NumInputs=6  Mode=Multidimensional array
  Selector : Selector  InputPortWidth=ROBOT_DOF+6  IndexOptions=Index vector (dialog)  Indices=[1:6]  OutputSizes=1
  Selector1 : Selector  InputPortWidth=ROBOT_DOF+6  IndexOptions=Index vector (dialog)  Indices=[7:ROBOT_DOF+6]  OutputSizes=1
  Vector Concatenate : Concatenate  NumInputs=6
  J_LFoot : Outport
  J_RFoot : Outport  Port=2
  J_CoM : Outport  Port=3
  J_rot_task : Outport  Port=4
  J_LHand : Outport  Port=5
  J_RHand : Outport  Port=6
  M : Outport  Port=7
  h : Outport  Port=8
  J : Outport  Port=9
  JDot_nu : Outport  Port=10
  wires:
  "               "/1 -> Vector Concatenate/4
  "  "/1 -> J_CoM/1, Matrix Concatenate/3
  "     "/1 -> J_rot_task/1, Matrix Concatenate/4
  Vector Concatenate/1 -> JDot_nu/1
  Selector1/1 -> Mass Matrix and Bias Forces/3(sDot), Jacobians and JDot_nu/3(sDot)
  nu/1 -> Selector/1, Selector1/1
  Selector/1 -> Mass Matrix and Bias Forces/2(nu_b), Jacobians and JDot_nu/2(nu_b)
  "   "/1 -> Vector Concatenate/3
  Mass Matrix and Bias Forces/2(M(q)) -> M/1
  Mass Matrix and Bias Forces/1(h(q,nu)) -> h/1
  s/1 -> Jacobians and JDot_nu/1(s), Mass Matrix and Bias Forces/1(s)
  w_H_b/1 -> Jacobians and JDot_nu/4(w_H_b), Mass Matrix and Bias Forces/4(w_H_b)
  Jacobians and JDot_nu/2(J_RFoot) -> J_RFoot/1, Matrix Concatenate/2
  Jacobians and JDot_nu/1(J_LFoot) -> J_LFoot/1, Matrix Concatenate/1
  Jacobians and JDot_nu/3(J_CoM) -> "  "/1
  Jacobians and JDot_nu/4(J_rot_task) -> "     "/1
  Jacobians and JDot_nu/7(JDot_nu_LFoot) -> Vector Concatenate/1
  Jacobians and JDot_nu/8(JDot_nu_RFoot) -> Vector Concatenate/2
  Jacobians and JDot_nu/9(JDot_nu_CoM) -> "   "/1
  Jacobians and JDot_nu/10(JDot_nu_rot_task) -> "               "/1
  Jacobians and JDot_nu/5(J_LHand) -> Matrix Concatenate/5, J_LHand/1
  Jacobians and JDot_nu/6(J_RHand) -> Matrix Concatenate/6, J_RHand/1
  Jacobians and JDot_nu/11(JDot_nu_LHand) -> Vector Concatenate/5
  Jacobians and JDot_nu/12(JDot_nu_RHand) -> Vector Concatenate/6
  Matrix Concatenate/1 -> J/1

== system torqueWalkingR2012b/Dynamics and Kinematics/Initial Conditions ==
  feetInContact : Inport
  s_sDot_sDDot_ref : Inport  Port=2
  "   1" : WBToolboxLibrary/Utilities/holder 
  "   2" : WBToolboxLibrary/Utilities/holder 
  Compute world to base transform : Subsystem
  Mux : Mux  Inputs=2
  Reshape : Reshape
  Selector : Selector  NumberOfDimensions=2  InputPortWidth=3  IndexOptions=Index vector (dialog),Index vector (dialog)  Indices=[1:ROBOT_DOF],1  OutputSizes=1,1
  Selector1 : Selector  NumberOfDimensions=2  InputPortWidth=3  IndexOptions=Index vector (dialog),Index vector (dialog)  Indices=[1:ROBOT_DOF],2  OutputSizes=1,1
  compute state velocity : Subsystem
  q_0 : Outport
  nu_0 : Outport  Port=2
  wires:
  Reshape/1 -> Mux/1
  Mux/1 -> q_0/1
  s_sDot_sDDot_ref/1 -> "   2"/1
  "   2"/1 -> Selector/1, Selector1/1
  Selector/1 -> Mux/2, compute state velocity/1(s), Compute world to base transform/1(s)
  compute state velocity/1(nu) -> nu_0/1
  feetInContact/1 -> "   1"/1
  Compute world to base transform/1(w_H_b) -> Reshape/1, compute state velocity/2(w_H_b)
  "   1"/1 -> compute state velocity/3("feetInContact ")
  Selector1/1 -> compute state velocity/4(sDot)

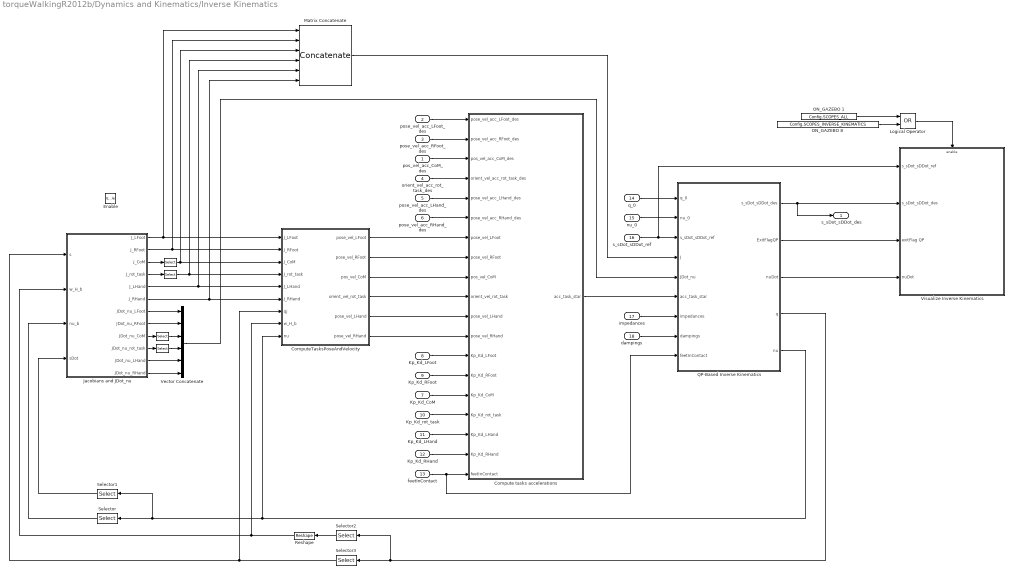
== system torqueWalkingR2012b/Dynamics and Kinematics/Inverse Kinematics ==
  pos_vel_acc_CoM_des : Inport
  pose_vel_acc_LFoot_des : Inport  Port=2
  pose_vel_acc_RFoot_des : Inport  Port=3
  orient_vel_acc_rot_task_des : Inport  Port=4
  pose_vel_acc_LHand_des : Inport  Port=5
  pose_vel_acc_RHand_des : Inport  Port=6
  Kp_Kd_CoM : Inport  Port=7
  Kp_Kd_LFoot : Inport  Port=8
  Kp_Kd_RFoot : Inport  Port=9
  Kp_Kd_rot_task : Inport  Port=10
  Kp_Kd_LHand : Inport  Port=11
  Kp_Kd_RHand : Inport  Port=12
  feetInContact : Inport  Port=13
  q_0 : Inport  Port=14
  nu_0 : Inport  Port=15
  s_sDot_sDDot_ref : Inport  Port=16
  impedances : Inport  Port=17
  dampings : Inport  Port=18
  Enable : EnablePort
  "  " : Selector  NumberOfDimensions=2  InputPortWidth=ROBOT_DOF+16  IndexOptions=Index vector (dialog),Index vector (dialog)  Indices=[1:3],[1:ROBOT_DOF+6]  OutputSizes=1,1
  "   " : Selector  InputPortWidth=6  IndexOptions=Index vector (dialog)  Indices=[1:3]  OutputSizes=1
  "     " : Selector  NumberOfDimensions=2  InputPortWidth=ROBOT_DOF+16  IndexOptions=Index vector (dialog),Index vector (dialog)  Indices=[4:6],[1:ROBOT_DOF+6]  OutputSizes=1,1
  "               " : Selector  InputPortWidth=6  IndexOptions=Index vector (dialog)  Indices=[4:6]  OutputSizes=1
  Compute tasks accelerations : MATLAB Function  TreatAsAtomicUnit=on
      settings: PermitHierarchicalResolution=ParametersOnly
  ComputeTasksPoseAndVelocity : Subsystem
  Jacobians and JDot_nu : Subsystem
  Logical Operator : Logic  Operator=OR  AllPortsSameDT=off  OutDataTypeStr=boolean
  Matrix Concatenate : Concatenate  NumInputs=6  Mode=Multidimensional array
  ON_GAZEBO 1 : Constant  Value=Config.SCOPES_ALL
  ON_GAZEBO 8 : Constant  Value=Config.SCOPES_INVERSE_KINEMATICS
  QP-Based Inverse Kinematics : Subsystem
  Reshape : Reshape  OutputDimensionality=Customize  OutputDimensions=[4,4]
  Selector : Selector  InputPortWidth=ROBOT_DOF+6  IndexOptions=Index vector (dialog)  Indices=[1:6]  OutputSizes=1
  Selector1 : Selector  InputPortWidth=ROBOT_DOF+6  IndexOptions=Index vector (dialog)  Indices=[7:ROBOT_DOF+6]  OutputSizes=1
  Selector2 : Selector  InputPortWidth=ROBOT_DOF+16  IndexOptions=Index vector (dialog)  Indices=[1:16]  OutputSizes=1
  Selector3 : Selector  InputPortWidth=ROBOT_DOF+16  IndexOptions=Index vector (dialog)  Indices=[17:ROBOT_DOF+16]  OutputSizes=1
  Vector Concatenate : Concatenate  NumInputs=6
  Visualize Inverse Kinematics : Subsystem
  s_sDot_sDDot_des : Outport
  wires:
  Kp_Kd_CoM/1 -> Compute tasks accelerations/15(Kp_Kd_CoM)
  Kp_Kd_LFoot/1 -> Compute tasks accelerations/13(Kp_Kd_LFoot)
  pose_vel_acc_LFoot_des/1 -> Compute tasks accelerations/1(pose_vel_acc_LFoot_des)
  Kp_Kd_RFoot/1 -> Compute tasks accelerations/14(Kp_Kd_RFoot)
  orient_vel_acc_rot_task_des/1 -> Compute tasks accelerations/4(orient_vel_acc_rot_task_des)
  pose_vel_acc_RFoot_des/1 -> Compute tasks accelerations/2(pose_vel_acc_RFoot_des)
  Kp_Kd_rot_task/1 -> Compute tasks accelerations/16(Kp_Kd_rot_task)
  pos_vel_acc_CoM_des/1 -> Compute tasks accelerations/3(pos_vel_acc_CoM_des)
  ComputeTasksPoseAndVelocity/3(pos_vel_CoM) -> Compute tasks accelerations/9(pos_vel_CoM)
  ComputeTasksPoseAndVelocity/1(pose_vel_LFoot) -> Compute tasks accelerations/7(pose_vel_LFoot)
  ComputeTasksPoseAndVelocity/2(pose_vel_RFoot) -> Compute tasks accelerations/8(pose_vel_RFoot)
  ComputeTasksPoseAndVelocity/4(orient_vel_rot_task) -> Compute tasks accelerations/10(orient_vel_rot_task)
  s_sDot_sDDot_ref/1 -> Visualize Inverse Kinematics/1(s_sDot_sDDot_ref), QP-Based Inverse Kinematics/3(s_sDot_sDDot_ref)
  Selector2/1 -> Reshape/1
  "  "/1 -> ComputeTasksPoseAndVelocity/3(J_CoM), Matrix Concatenate/3
  "   "/1 -> Vector Concatenate/3
  Jacobians and JDot_nu/2(J_RFoot) -> ComputeTasksPoseAndVelocity/2(J_RFoot), Matrix Concatenate/2
  Jacobians and JDot_nu/1(J_LFoot) -> ComputeTasksPoseAndVelocity/1(J_LFoot), Matrix Concatenate/1
  Selector1/1 -> Jacobians and JDot_nu/4(sDot)
  Selector/1 -> Jacobians and JDot_nu/3(nu_b)
  Jacobians and JDot_nu/4(J_rot_task) -> "     "/1
  Jacobians and JDot_nu/7(JDot_nu_LFoot) -> Vector Concatenate/1
  Jacobians and JDot_nu/8(JDot_nu_RFoot) -> Vector Concatenate/2
  Jacobians and JDot_nu/9(JDot_nu_CoM) -> "   "/1
  Jacobians and JDot_nu/10(JDot_nu_rot_task) -> "               "/1
  Vector Concatenate/1 -> QP-Based Inverse Kinematics/5(JDot_nu)
  dampings/1 -> QP-Based Inverse Kinematics/8(dampings)
  Compute tasks accelerations/1(acc_task_star) -> QP-Based Inverse Kinematics/6(acc_task_star)
  impedances/1 -> QP-Based Inverse Kinematics/7(impedances)
  Matrix Concatenate/1 -> QP-Based Inverse Kinematics/4(J)
  nu_0/1 -> QP-Based Inverse Kinematics/2(nu_0)
  q_0/1 -> QP-Based Inverse Kinematics/1(q_0)
  QP-Based Inverse Kinematics/5(nu) -> ComputeTasksPoseAndVelocity/9(nu), Selector1/1, Selector/1
  QP-Based Inverse Kinematics/4(q) -> Selector2/1, Selector3/1
  QP-Based Inverse Kinematics/1(s_sDot_sDDot_des) -> s_sDot_sDDot_des/1, Visualize Inverse Kinematics/2(s_sDot_sDDot_des)
  "     "/1 -> ComputeTasksPoseAndVelocity/4(J_rot_task), Matrix Concatenate/4
  "               "/1 -> Vector Concatenate/4
  Jacobians and JDot_nu/3(J_CoM) -> "  "/1
  Reshape/1 -> ComputeTasksPoseAndVelocity/8(w_H_b), Jacobians and JDot_nu/2(w_H_b)
  Selector3/1 -> ComputeTasksPoseAndVelocity/7(qj), Jacobians and JDot_nu/1(s)
  ON_GAZEBO 8/1 -> Logical Operator/2
  ON_GAZEBO 1/1 -> Logical Operator/1
  Logical Operator/1 -> Visualize Inverse Kinematics/Enable
  QP-Based Inverse Kinematics/2(ExitFlagQP) -> Visualize Inverse Kinematics/3(exitFlag QP)
  QP-Based Inverse Kinematics/3(nuDot) -> Visualize Inverse Kinematics/4(nuDot)
  Jacobians and JDot_nu/5(J_LHand) -> ComputeTasksPoseAndVelocity/5(J_LHand), Matrix Concatenate/5
  Jacobians and JDot_nu/6(J_RHand) -> ComputeTasksPoseAndVelocity/6(J_RHand), Matrix Concatenate/6
  Kp_Kd_LHand/1 -> Compute tasks accelerations/17(Kp_Kd_LHand)
  Kp_Kd_RHand/1 -> Compute tasks accelerations/18(Kp_Kd_RHand)
  ComputeTasksPoseAndVelocity/5(pose_vel_LHand) -> Compute tasks accelerations/11(pose_vel_LHand)
  ComputeTasksPoseAndVelocity/6(pose_vel_RHand) -> Compute tasks accelerations/12(pose_vel_RHand)
  pose_vel_acc_LHand_des/1 -> Compute tasks accelerations/5(pose_vel_acc_LHand_des)
  pose_vel_acc_RHand_des/1 -> Compute tasks accelerations/6(pose_vel_acc_RHand_des)
  Jacobians and JDot_nu/12(JDot_nu_RHand) -> Vector Concatenate/6
  Jacobians and JDot_nu/11(JDot_nu_LHand) -> Vector Concatenate/5
  feetInContact/1 -> QP-Based Inverse Kinematics/9(feetInContact), Compute tasks accelerations/19(feetInContact)

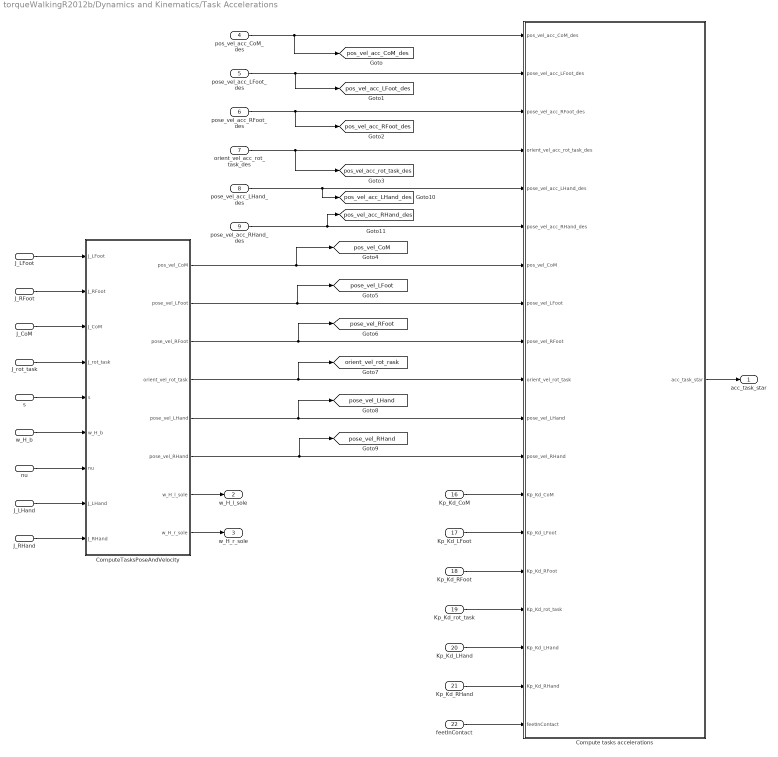
== system torqueWalkingR2012b/Dynamics and Kinematics/Task Accelerations ==
  s : Inport
  w_H_b : Inport  Port=2
  nu : Inport  Port=3
  pos_vel_acc_CoM_des : Inport  Port=4
  pose_vel_acc_LFoot_des : Inport  Port=5
  pose_vel_acc_RFoot_des : Inport  Port=6
  orient_vel_acc_rot_task_des : Inport  Port=7
  pose_vel_acc_LHand_des : Inport  Port=8
  pose_vel_acc_RHand_des : Inport  Port=9
  J_LFoot : Inport  Port=10
  J_RFoot : Inport  Port=11
  J_CoM : Inport  Port=12
  J_rot_task : Inport  Port=13
  J_LHand : Inport  Port=14
  J_RHand : Inport  Port=15
  Kp_Kd_CoM : Inport  Port=16
  Kp_Kd_LFoot : Inport  Port=17
  Kp_Kd_RFoot : Inport  Port=18
  Kp_Kd_rot_task : Inport  Port=19
  Kp_Kd_LHand : Inport  Port=20
  Kp_Kd_RHand : Inport  Port=21
  feetInContact : Inport  Port=22
  Compute tasks accelerations : MATLAB Function  TreatAsAtomicUnit=on
      settings: PermitHierarchicalResolution=ParametersOnly
  ComputeTasksPoseAndVelocity : Subsystem
  acc_task_star : Outport
  w_H_l_sole : Outport  Port=2
  w_H_r_sole : Outport  Port=3
  tag scope: orient_vel_rot_rask=global, pos_vel_CoM=global, pos_vel_acc_CoM_des=global, pos_vel_acc_LFoot_des=global, pos_vel_acc_LHand_des=global, pos_vel_acc_RFoot_des=global, pos_vel_acc_RHand_des=global, pos_vel_acc_rot_task_des=global, pose_vel_LFoot=global, pose_vel_LHand=global, pose_vel_RFoot=global, pose_vel_RHand=global
  wires:
  pos_vel_acc_CoM_des/1 -> [pos_vel_acc_CoM_des], Compute tasks accelerations/1(pos_vel_acc_CoM_des)
  Kp_Kd_RFoot/1 -> Compute tasks accelerations/15(Kp_Kd_RFoot)
  Kp_Kd_rot_task/1 -> Compute tasks accelerations/16(Kp_Kd_rot_task)
  feetInContact/1 -> Compute tasks accelerations/19(feetInContact)
  pose_vel_acc_RFoot_des/1 -> [pos_vel_acc_RFoot_des], Compute tasks accelerations/3(pose_vel_acc_RFoot_des)
  Kp_Kd_LFoot/1 -> Compute tasks accelerations/14(Kp_Kd_LFoot)
  Kp_Kd_CoM/1 -> Compute tasks accelerations/13(Kp_Kd_CoM)
  orient_vel_acc_rot_task_des/1 -> [pos_vel_acc_rot_task_des], Compute tasks accelerations/4(orient_vel_acc_rot_task_des)
  pose_vel_acc_LFoot_des/1 -> Compute tasks accelerations/2(pose_vel_acc_LFoot_des), [pos_vel_acc_LFoot_des]
  Compute tasks accelerations/1(acc_task_star) -> acc_task_star/1
  ComputeTasksPoseAndVelocity/1(pos_vel_CoM) -> [pos_vel_CoM], Compute tasks accelerations/7(pos_vel_CoM)
  ComputeTasksPoseAndVelocity/4(orient_vel_rot_task) -> Compute tasks accelerations/10(orient_vel_rot_task), [orient_vel_rot_rask]
  J_LFoot/1 -> ComputeTasksPoseAndVelocity/1(J_LFoot)
  J_RFoot/1 -> ComputeTasksPoseAndVelocity/2(J_RFoot)
  J_CoM/1 -> ComputeTasksPoseAndVelocity/3(J_CoM)
  J_rot_task/1 -> ComputeTasksPoseAndVelocity/4(J_rot_task)
  s/1 -> ComputeTasksPoseAndVelocity/5(s)
  w_H_b/1 -> ComputeTasksPoseAndVelocity/6(w_H_b)
  nu/1 -> ComputeTasksPoseAndVelocity/7(nu)
  ComputeTasksPoseAndVelocity/2(pose_vel_LFoot) -> Compute tasks accelerations/8(pose_vel_LFoot), [pose_vel_LFoot]
  ComputeTasksPoseAndVelocity/3(pose_vel_RFoot) -> Compute tasks accelerations/9(pose_vel_RFoot), [pose_vel_RFoot]
  ComputeTasksPoseAndVelocity/7(w_H_l_sole) -> w_H_l_sole/1
  ComputeTasksPoseAndVelocity/8(w_H_r_sole) -> w_H_r_sole/1
  J_RHand/1 -> ComputeTasksPoseAndVelocity/9(J_RHand)
  J_LHand/1 -> ComputeTasksPoseAndVelocity/8(J_LHand)
  ComputeTasksPoseAndVelocity/5(pose_vel_LHand) -> [pose_vel_LHand], Compute tasks accelerations/11(pose_vel_LHand)
  ComputeTasksPoseAndVelocity/6(pose_vel_RHand) -> [pose_vel_RHand], Compute tasks accelerations/12(pose_vel_RHand)
  pose_vel_acc_RHand_des/1 -> [pos_vel_acc_RHand_des], Compute tasks accelerations/6(pose_vel_acc_RHand_des)
  pose_vel_acc_LHand_des/1 -> [pos_vel_acc_LHand_des], Compute tasks accelerations/5(pose_vel_acc_LHand_des)
  Kp_Kd_RHand/1 -> Compute tasks accelerations/18(Kp_Kd_RHand)
  Kp_Kd_LHand/1 -> Compute tasks accelerations/17(Kp_Kd_LHand)

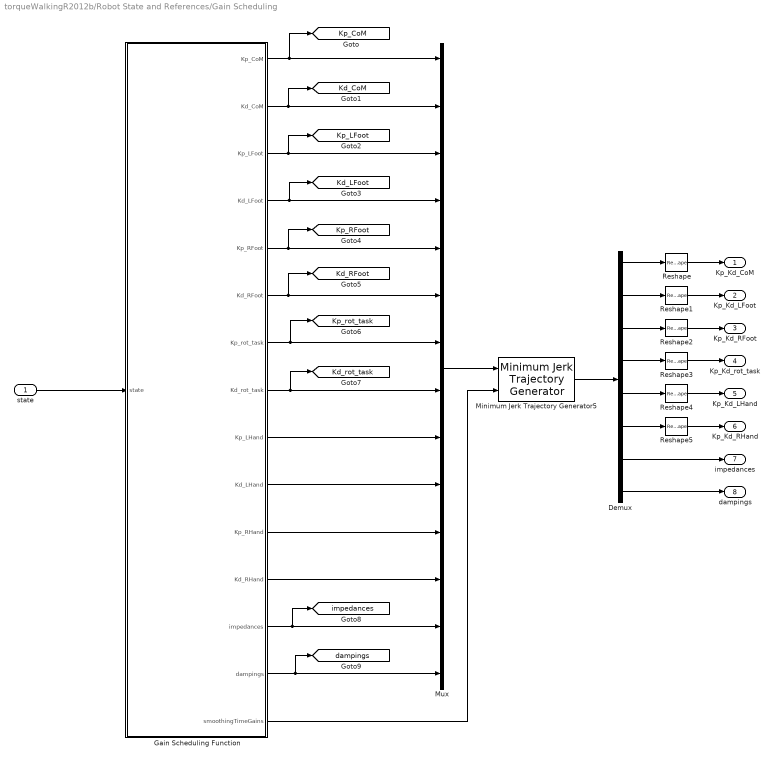
== system torqueWalkingR2012b/Robot State and References/Gain Scheduling ==
  state : Inport
  Demux : Demux  Outputs=[6;12;12;6;12;12;ROBOT_DOF;ROBOT_DOF]
  Gain Scheduling Function : MATLAB Function  TreatAsAtomicUnit=on
      settings: PermitHierarchicalResolution=ParametersOnly
  Minimum Jerk Trajectory Generator5 : WBToolboxLibrary/Utilities/Minimum Jerk Trajectory Generator  externalSettlingTime=on  settlingTime=3  sampleTime=Config.t_step  resetOnSettlingTime=off  firstDerivatives=off  secondDerivatives=off  explicitInitialValue=off
  Mux : Mux  Inputs=14
  Reshape : Reshape  OutputDimensionality=Customize  OutputDimensions=[3;2]
  Reshape{1..2,4..5} (4 alike) : Reshape  OutputDimensionality=Customize  OutputDimensions=[6;2]
  Reshape3 : Reshape  OutputDimensionality=Customize  OutputDimensions=[3;2]
  Kp_Kd_CoM : Outport
  Kp_Kd_LFoot : Outport  Port=2
  Kp_Kd_RFoot : Outport  Port=3
  Kp_Kd_rot_task : Outport  Port=4
  Kp_Kd_LHand : Outport  Port=5
  Kp_Kd_RHand : Outport  Port=6
  impedances : Outport  Port=7
  dampings : Outport  Port=8
  tag scope: Kd_CoM=global, Kd_LFoot=global, Kd_RFoot=global, Kd_rot_task=global, Kp_CoM=global, Kp_LFoot=global, Kp_RFoot=global, Kp_rot_task=global, dampings=global, impedances=global
  wires:
  state/1 -> Gain Scheduling Function/1(state)
  Gain Scheduling Function/1(Kp_CoM) -> [Kp_CoM], Mux/1
  Gain Scheduling Function/2(Kd_CoM) -> [Kd_CoM], Mux/2
  Gain Scheduling Function/3(Kp_LFoot) -> [Kp_LFoot], Mux/3
  Gain Scheduling Function/4(Kd_LFoot) -> [Kd_LFoot], Mux/4
  Gain Scheduling Function/5(Kp_RFoot) -> [Kp_RFoot], Mux/5
  Gain Scheduling Function/6(Kd_RFoot) -> [Kd_RFoot], Mux/6
  Gain Scheduling Function/7(Kp_rot_task) -> [Kp_rot_task], Mux/7
  Gain Scheduling Function/8(Kd_rot_task) -> [Kd_rot_task], Mux/8
  Mux/1 -> Minimum Jerk Trajectory Generator5/1
  Gain Scheduling Function/13(impedances) -> Mux/13, [impedances]
  Gain Scheduling Function/14(dampings) -> [dampings], Mux/14
  Gain Scheduling Function/15(smoothingTimeGains) -> Minimum Jerk Trajectory Generator5/2
  Minimum Jerk Trajectory Generator5/1 -> Demux/1
  Demux/1 -> Reshape/1
  Demux/2 -> Reshape1/1
  Demux/3 -> Reshape2/1
  Demux/4 -> Reshape3/1
  Reshape/1 -> Kp_Kd_CoM/1
  Reshape1/1 -> Kp_Kd_LFoot/1
  Reshape2/1 -> Kp_Kd_RFoot/1
  Reshape3/1 -> Kp_Kd_rot_task/1
  Demux/7 -> impedances/1
  Demux/8 -> dampings/1
  Gain Scheduling Function/9(Kp_LHand) -> Mux/9
  Gain Scheduling Function/10(Kd_LHand) -> Mux/10
  Gain Scheduling Function/11(Kp_RHand) -> Mux/11
  Gain Scheduling Function/12(Kd_RHand) -> Mux/12
  Reshape5/1 -> Kp_Kd_RHand/1
  Reshape4/1 -> Kp_Kd_LHand/1
  Demux/6 -> Reshape5/1
  Demux/5 -> Reshape4/1

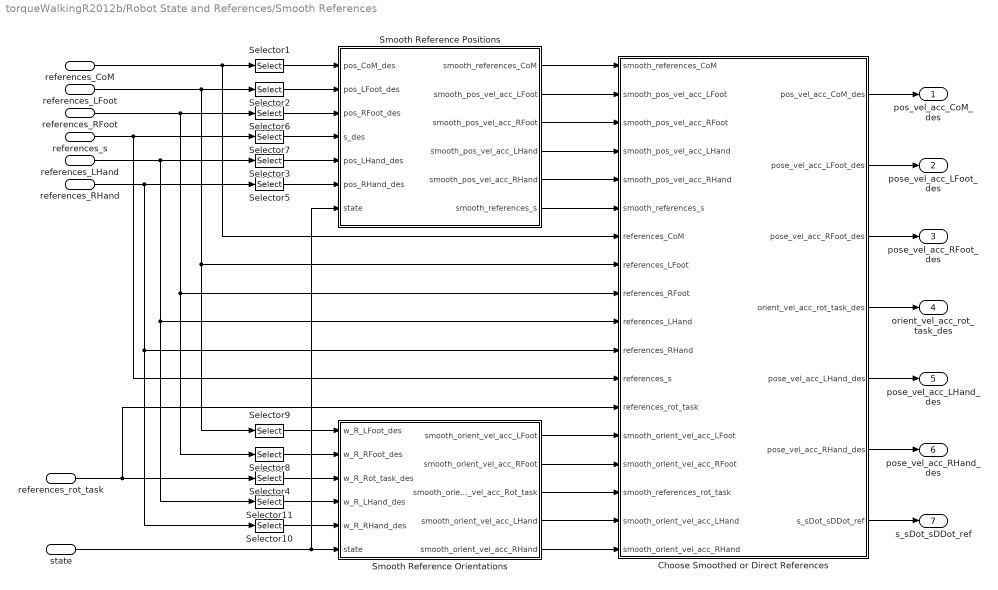
== system torqueWalkingR2012b/Robot State and References/Smooth References  ==
  state : Inport
  references_LFoot : Inport  Port=2
  references_RFoot : Inport  Port=3
  references_CoM : Inport  Port=4
  references_rot_task : Inport  Port=5
  references_LHand : Inport  Port=6
  references_RHand : Inport  Port=7
  references_s : Inport  Port=8
  Choose Smoothed or Direct References : Subsystem
  Selector{1..3,5..6} (5 alike) : Selector  NumberOfDimensions=2  InputPortWidth=3  IndexOptions=Index vector (dialog),Index vector (dialog)  Indices=[1:3],1  OutputSizes=1,1
  Selector{8..11} (4 alike) : Selector  NumberOfDimensions=2  InputPortWidth=3  IndexOptions=Index vector (dialog),Index vector (dialog)  Indices=[4:6],[1:3]  OutputSizes=1,1
  Selector4 : Selector  NumberOfDimensions=2  InputPortWidth=3  IndexOptions=Index vector (dialog),Index vector (dialog)  Indices=[1:3],[1:3]  OutputSizes=1,1
  Selector7 : Selector  NumberOfDimensions=2  InputPortWidth=ROBOT_DOF  IndexOptions=Index vector (dialog),Index vector (dialog)  Indices=[1:ROBOT_DOF],1  OutputSizes=1,1
  Smooth Reference Orientations : Subsystem
  Smooth Reference Positions : Subsystem
  pos_vel_acc_CoM_des : Outport
  pose_vel_acc_LFoot_des : Outport  Port=2
  pose_vel_acc_RFoot_des : Outport  Port=3
  orient_vel_acc_rot_task_des : Outport  Port=4
  pose_vel_acc_LHand_des : Outport  Port=5
  pose_vel_acc_RHand_des : Outport  Port=6
  s_sDot_sDDot_ref : Outport  Port=7
  wires:
  references_CoM/1 -> Choose Smoothed or Direct References/7(references_CoM), Selector1/1
  Selector1/1 -> Smooth Reference Positions/1(pos_CoM_des)
  references_LFoot/1 -> Choose Smoothed or Direct References/8(references_LFoot), Selector9/1, Selector2/1
  Selector2/1 -> Smooth Reference Positions/2(pos_LFoot_des)
  references_RFoot/1 -> Selector8/1, Choose Smoothed or Direct References/9(references_RFoot), Selector6/1
  Selector6/1 -> Smooth Reference Positions/3(pos_RFoot_des)
  references_s/1 -> Selector7/1, Choose Smoothed or Direct References/12(references_s)
  Selector7/1 -> Smooth Reference Positions/4(s_des)
  references_rot_task/1 -> Selector4/1, Choose Smoothed or Direct References/13(references_rot_task)
  Selector4/1 -> Smooth Reference Orientations/3(w_R_Rot_task_des)
  Selector8/1 -> Smooth Reference Orientations/2(w_R_RFoot_des)
  Selector9/1 -> Smooth Reference Orientations/1(w_R_LFoot_des)
  Smooth Reference Positions/1(smooth_references_CoM) -> Choose Smoothed or Direct References/1(smooth_references_CoM)
  Smooth Reference Orientations/3(smooth_orient_vel_acc_Rot_task) -> Choose Smoothed or Direct References/16(smooth_references_rot_task)
  Smooth Reference Orientations/2(smooth_orient_vel_acc_RFoot) -> Choose Smoothed or Direct References/15(smooth_orient_vel_acc_RFoot)
  Smooth Reference Orientations/1(smooth_orient_vel_acc_LFoot) -> Choose Smoothed or Direct References/14(smooth_orient_vel_acc_LFoot)
  Choose Smoothed or Direct References/1(pos_vel_acc_CoM_des) -> pos_vel_acc_CoM_des/1
  Choose Smoothed or Direct References/2(pose_vel_acc_LFoot_des) -> pose_vel_acc_LFoot_des/1
  Choose Smoothed or Direct References/7(s_sDot_sDDot_ref) -> s_sDot_sDDot_ref/1
  Choose Smoothed or Direct References/4(orient_vel_acc_rot_task_des) -> orient_vel_acc_rot_task_des/1
  Choose Smoothed or Direct References/3(pose_vel_acc_RFoot_des) -> pose_vel_acc_RFoot_des/1
  state/1 -> Smooth Reference Positions/7(state), Smooth Reference Orientations/6(state)
  Smooth Reference Positions/2(smooth_pos_vel_acc_LFoot) -> Choose Smoothed or Direct References/2(smooth_pos_vel_acc_LFoot)
  Smooth Reference Positions/3(smooth_pos_vel_acc_RFoot) -> Choose Smoothed or Direct References/3(smooth_pos_vel_acc_RFoot)
  Smooth Reference Positions/6(smooth_references_s) -> Choose Smoothed or Direct References/6(smooth_references_s)
  Selector3/1 -> Smooth Reference Positions/5(pos_LHand_des)
  references_LHand/1 -> Selector3/1, Selector11/1, Choose Smoothed or Direct References/10(references_LHand)
  Selector5/1 -> Smooth Reference Positions/6(pos_RHand_des)
  references_RHand/1 -> Selector5/1, Selector10/1, Choose Smoothed or Direct References/11(references_RHand)
  Smooth Reference Positions/4(smooth_pos_vel_acc_LHand) -> Choose Smoothed or Direct References/4(smooth_pos_vel_acc_LHand)
  Smooth Reference Positions/5(smooth_pos_vel_acc_RHand) -> Choose Smoothed or Direct References/5(smooth_pos_vel_acc_RHand)
  Selector11/1 -> Smooth Reference Orientations/4(w_R_LHand_des)
  Selector10/1 -> Smooth Reference Orientations/5(w_R_RHand_des)
  Smooth Reference Orientations/4(smooth_orient_vel_acc_LHand) -> Choose Smoothed or Direct References/17(smooth_orient_vel_acc_LHand)
  Smooth Reference Orientations/5(smooth_orient_vel_acc_RHand) -> Choose Smoothed or Direct References/18(smooth_orient_vel_acc_RHand)
  Choose Smoothed or Direct References/5(pose_vel_acc_LHand_des) -> pose_vel_acc_LHand_des/1
  Choose Smoothed or Direct References/6(pose_vel_acc_RHand_des) -> pose_vel_acc_RHand_des/1
